simulink model "exc1_"  (R2024b)
settings: Solver=FixedStepAuto  StartTime=0.0  StopTime=10.0  FixedStep=1  RelTol=1e-3
settings Model: Creator=ramse  LastModifiedBy=ramse

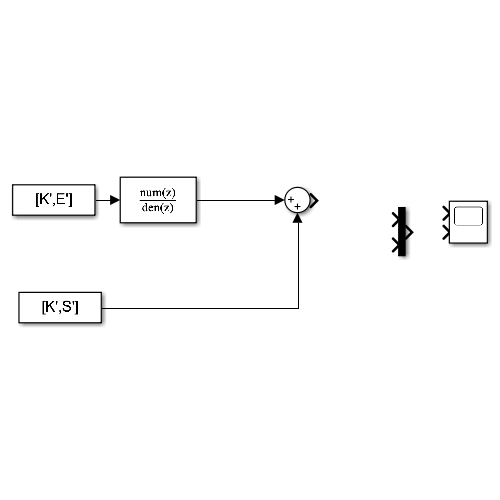
[thumbnail: Simulink's stored preview of the top-level diagram]
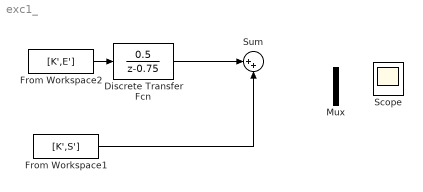
== system exc1_ ==
  Discrete Transfer Fcn : DiscreteTransferFcn  Numerator=[0.5]  Denominator=[1 -0.75]
  From Workspace1 : FromWorkspace  VariableName=[K',S']
  From Workspace2 : FromWorkspace  VariableName=[K',E']
  Mux : Mux  Inputs=2
  Scope : Scope  NumInputPorts=2
  Sum : Sum  Inputs=|++
  wires:
  From Workspace1/1 -> Sum/2
  From Workspace2/1 -> Discrete Transfer Fcn/1
  Discrete Transfer Fcn/1 -> Sum/1
